simulink library "pil"  (Simulink 3.00)
undefined symbols (not defined in the file or in its folder): j
libraries: smxl x70, SMXL x16
settings Model: LastModifiedBy=campa

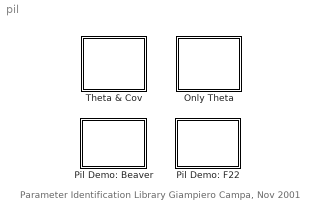
== system pil ==
  note: Parameter Identification Library
      | Giampiero Campa, Nov 2001
  Only Theta : Subsystem
  Pil Demo: Beaver : Subsystem
      settings: OpenFcn=beapilpath=which('pil');path(path,[ beapilpath(1:length(beapilpath)-8) '\examples' ]);clear beapilpath; load beadata; beapil;
      mask Display: disp('Beaver PIL\nDemo')
  Pil Demo: F22 : Subsystem
      settings: OpenFcn=f22pilpath=which('pil');path(path,[ f22pilpath(1:length(f22pilpath)-8) '\examples' ]);clear f22pilpath; load f22data; f22pil;
      mask Display: disp('F22 PIL\nDemo')
  Theta & Cov : Subsystem

== system pil/Only Theta ==
  FTR : Subsystem  mask(Fourier Transform Regression){ths=[4 2], w=2*pi*linspace(0.02,1.8,32)', T=0.025}
      mask prompts: ths "Theta Size"; w "Omega Points"; T "Sample Time"
      mask help:
      | This block performs FTR on the equation :
      |           E*zdot  +  F*z  =  x*TH
      |   The three inputs are respectively x,  E*z, F*z.
      |   The outputs is TH.
      |   The FTR is performed along the points of the omega
      |   vector supplied as the second mask parameter.
      |   The Derivative od E*z is taken by multiplying
      |   its fourier transform by jw.
      mask init:
      | n=length(w);m=ths(1);p=ths(2);
      mask Help:
      | This block performs FTR on the equation :
      |           E*zdot  +  F*z  =  x*TH
      |   The three inputs are respectively x,  E*z, F*z.
      |   The two outputs is TH.
      |   The FTR is performed along the points of the omega
      |   vector supplied as the second mask parameter.
      |   The Derivative od E*z is taken by multiplying
      |   its fourier transform by jw.
      | 
      |   Due to the sampling theorem, for the FT to make
      |   sense the following 2 equations should be valid :
      |   4*pi*wmax*T         <  1 ,
      |   4*pi*Tsim*wmin     >  1 .
      | 
      |   This block needs the Simulink Matrix Library.
  FTR-TD : Subsystem  mask(Fourier Transform Regression (derivative in Time Domain)){ths=[4 2], w=2*pi*linspace(0.02,1.8,32)', T=0.025}
      mask prompts: ths "Theta Size"; w "Omega Points"; T "Sample Time"
      mask help:
      | This block performs FTR on the equation :
      |           E*zdot  +  F*z  =  x*TH
      |   The three inputs are respectively x,  E*z, F*z.
      |   The output is TH.
      |   The FTR is performed along the points of the omega
      |   vector supplied as the second mask parameter.
      |   The Derivative od E*z is taken in the time domain
      |   with the respective simulink block.
      mask init:
      | n=length(w);m=ths(1);p=ths(2);
      mask Help:
      | This block performs FTR on the equation :
      |           E*zdot  +  F*z  =  x*TH
      |   The three inputs are respectively x,  E*z, F*z.
      |   The output is TH.
      |   The FTR is performed along the points of the omega
      |   vector supplied as the second mask parameter.
      |   The Derivative od E*z is taken in the time domain
      |   with the respective simulink block.
      | 
      |   Due to the sampling theorem, for the FT to make
      |   sense the following 2 equations should be valid :
      |   4*pi*wmax*T         <  1 ,
      |   4*pi*Tsim*wmin     >  1 .
      | 
      |   While TH could be of any size, the covariance matrix
      |   is the actual one only if theta is a column vector,
      |   otherwise it's just an approximation of the mean covariance
      |   matrix between the covariance matrices of the different
      |   column vectors that compose TH.
      | 
      |   This block needs the Simulink Matrix Library.
  LLS : Subsystem  mask(Local Least Square){ths=[4 2], n=50, T=0.025}
      mask prompts: ths "Theta Size"; n "Window Size"; T "Sample Time"
      mask help:
      | This block performs LLS on the equation :
      |           E*zdot  +  F*z  =  x*TH
      |   The three inputs are respectively x,  E*z, F*z.
      |   The window size is supplied as a mask parameter.
      mask init:
      | m=ths(1);p=ths(2);
      mask Help:
      | This block performs LLS on the equation :
      |           E*zdot  +  F*z  =  x*TH
      |   The three inputs are respectively x,  E*z, F*z.
      |   The window size is supplied as a mask parameter.
      | 
      |   This block needs the Simulink Matrix Library.
  NRLS : Subsystem  mask(Normalized Recursive Least Squares Regression){ths=[4 2], lam=.9, T=0.025}
      mask prompts: ths "Theta Size"; lam "Forgetting Factor"; T "Sample Time"
      mask help:
      | This block performs NRLS on the equation :
      |           E*zdot  +  F*z  =  x*TH
      |   The three inputs are respectively x,  E*z, F*z.
      |   The outputs is TH.
      |   The forgetting factor is supplied as mask parameter.
      mask init:
      | m=ths(1);p=ths(2);
      mask Help:
      | This block performs RLS on the equation :
      |           E*zdot  +  F*z  =  x*TH
      |   The three inputs are respectively x,  E*z, F*z.
      |   The outputs is TH.
      |   The forgetting factor is supplied as mask parameter.
      | 
      |   This block needs the Simulink Matrix Library.
  RLS : Subsystem  mask(Recursive Least Square Regression){ths=[4 2], lam=.9, T=0.025}
      mask prompts: ths "Theta Size"; lam "Forgetting Factor"; T "Sample Time"
      mask help:
      | This block performs RLS on the equation :
      |           E*zdot  +  F*z  =  x*TH
      |   The three inputs are respectively x,  E*z, F*z.
      |   The outputs is TH.
      |   The forgetting factor is supplied as mask parameter.
      mask init:
      | m=ths(1);p=ths(2);
      mask Help:
      | This block performs RLS on the equation :
      |           E*zdot  +  F*z  =  x*TH
      |   The three inputs are respectively x,  E*z, F*z.
      |   The outputs is TH.
      |   The forgetting factor is supplied as mask parameter.
      | 
      |   This block needs the Simulink Matrix Library.

== system pil/Pil Demo: Beaver ==

== system pil/Pil Demo: F22 ==

== system pil/Theta & Cov ==
  FTR : Subsystem  mask(Fourier Transform Regression){ths=[4 2], w=2*pi*linspace(0.02,1.8,32)', T=0.025}
      mask prompts: ths "Theta Size"; w "Omega Points"; T "Sample Time"
      mask help:
      | This block performs FTR on the equation :
      |           E*zdot  +  F*z  =  x*TH
      |   The three inputs are respectively x,  E*z, F*z.
      |   The two outputs are TH and its covariance matrix.
      |   The FTR is performed along the points of the omega
      |   vector supplied as the second mask parameter.
      |   The Derivative od E*z is taken by multiplying
      |   its fourier transform by jw.
      mask init:
      | n=length(w);m=ths(1);p=ths(2);
      mask Help:
      | This block performs FTR on the equation :
      |           E*zdot  +  F*z  =  x*TH
      |   The three inputs are respectively x,  E*z, F*z.
      |   The two outputs are TH and its covariance matrix.
      |   The FTR is performed along the points of the omega
      |   vector supplied as the second mask parameter.
      |   The Derivative od E*z is taken by multiplying
      |   its fourier transform by jw.
      | 
      |   Due to the sampling theorem, for the FT to make
      |   sense the following 2 equations should be valid :
      |   4*pi*wmax*T         <  1 ,
      |   4*pi*Tsim*wmin     >  1 .
      | 
      |   While TH could be of any size, the covariance matrix
      |   is the actual one only if theta is a column vector,
      |   otherwise it's just an approximation of the mean covariance
      |   matrix between the covariance matrices of the different
      |   column vectors that compose TH.
      | 
      |   This block needs the Simulink Matrix Library.
  FTR-TD : Subsystem  mask(Fourier Transform Regression (derivative in Time Domain)){ths=[4 2], w=2*pi*linspace(0.02,1.8,32)', T=0.025}
      mask prompts: ths "Theta Size"; w "Omega Points"; T "Sample Time"
      mask help:
      | This block performs FTR on the equation :
      |           E*zdot  +  F*z  =  x*TH
      |   The three inputs are respectively x,  E*z, F*z.
      |   The two outputs are TH and its covariance matrix.
      |   The FTR is performed along the points of the omega
      |   vector supplied as the second mask parameter.
      |   The Derivative od E*z is taken in the time domain
      |   with the respective simulink block.
      mask init:
      | n=length(w);m=ths(1);p=ths(2);
      mask Help:
      | This block performs FTR on the equation :
      |           E*zdot  +  F*z  =  x*TH
      |   The three inputs are respectively x,  E*z, F*z.
      |   The two outputs are TH and its covariance matrix.
      |   The FTR is performed along the points of the omega
      |   vector supplied as the second mask parameter.
      |   The Derivative od E*z is taken in the time domain
      |   with the respective simulink block.
      | 
      |   Due to the sampling theorem, for the FT to make
      |   sense the following 2 equations should be valid :
      |   4*pi*wmax*T         <  1 ,
      |   4*pi*Tsim*wmin     >  1 .
      | 
      |   While TH could be of any size, the covariance matrix
      |   is the actual one only if theta is a column vector,
      |   otherwise it's just an approximation of the mean covariance
      |   matrix between the covariance matrices of the different
      |   column vectors that compose TH.
      | 
      |   This block needs the Simulink Matrix Library.
  LWR : Subsystem  mask(Local Weighted Regression){ths=[4 2], n=50, sig=1, T=0.025}
      mask prompts: ths "Theta Size"; n "Window Size"; sig "Gaussian Width"; T "Sample Time"
      mask help:
      | This block performs LWR on the equation :
      |           E*zdot  +  F*z  =  x*TH
      |   The three inputs are respectively x,  E*z, F*z.
      |   The two outputs are TH and its covariance matrix.
      |   The window size and the gaussian width are supplied
      |   as mask parameters. The weighting matrix is diagonal
      |   with W(i,i) = exp(-(x(t)-row(x(t),i))*/(2*sig^2)).
      mask init:
      | m=ths(1);p=ths(2);
      mask Help:
      | This block performs LWR on the equation :
      |           E*zdot  +  F*z  =  x*TH
      |   The three inputs are respectively x,  E*z, F*z.
      |   The two outputs are TH and its covariance matrix.
      |   The window size and the gaussian width are supplied
      |   as mask parameters. The weighting matrix is diagonal
      |   with W(i,i) = exp(-(x(t)-row(x(t),i))*/(2*sig^2)).
      | 
      |   While TH could be of any size, the covariance matrix
      |   is the actual one only if theta is a column vector,
      |   otherwise it's just an approximation of the mean covariance
      |   matrix between the covariance matrices of the different
      |   column vectors that compose TH.
      | 
      |   This block needs the Simulink Matrix Library.
  LWR-RD : Subsystem  mask(Local Weighted Regression with Retention and Deletion){ths=[4 2], n=50, sig=1, Tol=1e-6, x0=1, T=0.025}
      mask prompts: ths "Theta Size"; n "Window Size"; sig "Gaussian Width (sigma)"; Tol "Tolerance (x<tol means x=0)"; x0 "x0 (X0=x0*rand(n,m+2*p))"; T "Sample Time"
      mask help:
      | This block performs LWR on the equation :
      |           E*zdot  +  F*z  =  x*TH
      |   The three inputs are respectively x,  E*z, F*z.
      |   The two outputs are TH and its covariance matrix.
      |   The window size and the gaussian width are supplied
      |   as mask parameters. The weighting matrix is diagonal
      |   with W(i,i) = exp(-(x(t)-row(x(t),i))*/(2*sigma^2)).
      mask init:
      | m=ths(1);p=ths(2);
      mask Help:
      | This block performs LWR on the equation :
      |           E*zdot  +  F*z  =  x*TH
      |   The three inputs are respectively x,  E*z, F*z.
      |   The two outputs are TH and its covariance matrix.
      |   The window size and the gaussian width are supplied
      |   as mask parameters. The weighting matrix is diagonal
      |   with W(i,i) = exp(-(x(t)-row(x(t),i))*/(2*sigma^2)).
      | 
      |   While TH could be of any size, the covariance matrix
      |   is the actual one only if theta is a column vector,
      |   otherwise it's just an approximation of the mean covariance
      |   matrix between the covariance matrices of the different
      |   column vectors that compose TH.
      | 
      |   This block needs the Simulink Matrix Library.
  LWR-RD (Matlab) : Subsystem  mask(Local Weighted Regression with Retention and Deletion){ths=[4 2], n=50, sig=1, Tol=1e-6, T=0.025}
      mask prompts: ths "Theta Size"; n "Window Size"; sig "Gaussian Width (sigma)"; Tol "Tolerance (x<tol means x=0)"; T "Sample Time"
      mask help:
      | This block performs LWR on the equation :
      |           E*zdot  +  F*z  =  x*TH
      |   The three inputs are respectively x,  E*z, F*z.
      |   The two outputs are TH and its covariance matrix.
      |   The window size and the gaussian width are supplied
      |   as mask parameters. The weighting matrix is diagonal
      |   with W(i,i) = exp(-(x(t)-row(x(t),i))*/(2*sigma^2)).
      |   This version is based on the m-file s-function lwrb2.m,
      |   and it is therefore slightly slower than the normal version.
      mask init:
      | m=ths(1);p=ths(2);
      mask Help:
      | This block performs LWR on the equation :
      |           E*zdot  +  F*z  =  x*TH
      |   The three inputs are respectively x,  E*z, F*z.
      |   The two outputs are TH and its covariance matrix.
      |   The window size and the gaussian width are supplied
      |   as mask parameters. The weighting matrix is diagonal
      |   with W(i,i) = exp(-(x(t)-row(x(t),i))*/(2*sigma^2)).
      | 
      |   While TH could be of any size, the covariance matrix
      |   is the actual one only if theta is a column vector,
      |   otherwise it's just an approximation of the mean covariance
      |   matrix between the covariance matrices of the different
      |   column vectors that compose TH.
      | 
      |   This version is based on the m-file s-function lwrb2.m,
      |   and it is therefore slightly slower than the normal version.

== system pil/Only Theta/FTR ==
  x : Inport  Port=1  PortWidth=-1  SampleTime=-1  DataType=auto
      settings: SignalType=auto
  Ez : Inport  Port=2  PortWidth=-1  SampleTime=-1  DataType=auto
      settings: SignalType=auto
  Fz : Inport  Port=3  PortWidth=-1  SampleTime=-1  DataType=auto
      settings: SignalType=auto
  DTFT : Subsystem
  Demux2 : Demux  Outputs=[n*m n*p n*p]
  Mux : Mux  Inputs=[m p p]
  Regression : Subsystem
  Sum4 : Sum  Inputs=|++  SaturateOnIntegerOverflow=on
  jw : Gain  Gain=reshape(j*w*ones(1,p),n*p,1)  SaturateOnIntegerOverflow=on
  Theta : Outport  Port=1
  wires:
  DTFT/1(x(jw)) -> Demux2/1
  Demux2/2 -> jw/1
  Mux/1 -> DTFT/1(x(t))
  x/1 -> Mux/1
  Ez/1 -> Mux/2
  Fz/1 -> Mux/3
  Demux2/1 -> Regression/1(X)
  Demux2/3 -> Sum4/2
  jw/1 -> Sum4/1
  Sum4/1 -> Regression/2(Y)
  Regression/1(Theta) -> Theta/1

== system pil/Only Theta/FTR-TD ==
  x : Inport  Port=1  PortWidth=-1  SampleTime=-1  DataType=auto
      settings: SignalType=auto
  Ez : Inport  Port=2  PortWidth=-1  SampleTime=-1  DataType=auto
      settings: SignalType=auto
  Fz : Inport  Port=3  PortWidth=-1  SampleTime=-1  DataType=auto
      settings: SignalType=auto
  DTFT : Subsystem
  Demux2 : Demux  Outputs=[n*m n*p]
  Gain : Gain  Gain=1/T  SaturateOnIntegerOverflow=on
  Mux : Mux  Inputs=[m p]
  Regression : Subsystem
  Sum5 : Sum  Inputs=+-+  SaturateOnIntegerOverflow=on
  Unit Delay : UnitDelay  X0=zeros(p,1)  SampleTime=T
  Theta : Outport  Port=1
  wires:
  Sum5/1 -> Mux/2
  x/1 -> Mux/1
  Fz/1 -> Sum5/3
  Ez/1 -> Gain/1
  Gain/1 -> Sum5/1, Unit Delay/1
  Unit Delay/1 -> Sum5/2
  Demux2/2 -> Regression/2(Y)
  Demux2/1 -> Regression/1(X)
  Regression/1(Theta) -> Theta/1
  DTFT/1(x(jw)) -> Demux2/1
  Mux/1 -> DTFT/1(x(t))

== system pil/Only Theta/LLS ==
  x : Inport  Port=1  PortWidth=-1  SampleTime=-1  DataType=auto
      settings: SignalType=auto
  Ez : Inport  Port=2  PortWidth=-1  SampleTime=-1  DataType=auto
      settings: SignalType=auto
  Fz : Inport  Port=3  PortWidth=-1  SampleTime=-1  DataType=auto
      settings: SignalType=auto
  1/z Chain : Subsystem  mask(Discrete Time Brunowsky Form){ni=m+p, rd=n-1, x0=0, T=T}
      mask prompts: ni "Number of Inputs"; rd "Number of Delays for each Input"; x0 "Initial Condition"; T "Sample Time"
      mask help: Brunowsky Form System
      mask init:
      | a=[];b=[];c=[];d=[];
      | for i=1:ni,
      | a=[a,zeros(size(a,1),rd);zeros(rd,size(a,2)),diag(ones(rd-1,1),1)];
      | b=[b,zeros(size(b,1),1);zeros(rd,size(b,2)),[zeros(rd-1,1);1]];
      | c=[c,zeros(size(c,1),rd);zeros(rd+1,size(c,2)),[eye(rd);zeros(1,rd)]];
      | d=[d,zeros(size(d,1),1);zeros(rd+1,size(d,2)),[zeros(rd,1);1]];
      | end
      mask Help:
      | <p>
      | This block implements a Brunowsky Form System: every inputs passes through n delays.
      | </p>
      | Outputs are simply all the states of the system.
      mask Display: disp('1/z^n')
  Demux2 : Demux  Outputs=[n*m n*p]
  Gain : Gain  Gain=1/T  SaturateOnIntegerOverflow=on
  Mux : Mux  Inputs=[m p]
  Sum5 : Sum  Inputs=+-+  SaturateOnIntegerOverflow=on
  Unit Delay : UnitDelay  X0=zeros(p,1)  SampleTime=T
  vrmult2 : SMXL/Real Matrices/vrmult  dims=[m n p]
  vrpinv : SMXL/Real Matrices/vrpinv  dims=[n m]  tol=1
  Theta : Outport  Port=1
  wires:
  vrpinv/1 -> vrmult2/1
  vrmult2/1 -> Theta/1
  Mux/1 -> 1/z Chain/1(In)
  Demux2/1 -> vrpinv/1
  Demux2/2 -> vrmult2/2
  1/z Chain/1(Out) -> Demux2/1
  Sum5/1 -> Mux/2
  x/1 -> Mux/1
  Fz/1 -> Sum5/3
  Ez/1 -> Gain/1
  Gain/1 -> Sum5/1, Unit Delay/1
  Unit Delay/1 -> Sum5/2

== system pil/Only Theta/NRLS ==
  x : Inport  Port=1  PortWidth=-1  SampleTime=-1  DataType=auto
      settings: SignalType=auto
  Ez : Inport  Port=2  PortWidth=-1  SampleTime=-1  DataType=auto
      settings: SignalType=auto
  Fz : Inport  Port=3  PortWidth=-1  SampleTime=-1  DataType=auto
      settings: SignalType=auto
  Gain : Gain  Gain=1/T  SaturateOnIntegerOverflow=on
  Regression : Subsystem
  Sum5 : Sum  Inputs=+-+  SaturateOnIntegerOverflow=on
  Unit Delay : UnitDelay  X0=zeros(p,1)  SampleTime=T
  Theta : Outport  Port=1
  wires:
  Regression/1(Theta) -> Theta/1
  Sum5/1 -> Regression/2(Y)
  x/1 -> Regression/1(X)
  Fz/1 -> Sum5/3
  Ez/1 -> Gain/1
  Gain/1 -> Unit Delay/1, Sum5/1
  Unit Delay/1 -> Sum5/2

== system pil/Only Theta/RLS ==
  x : Inport  Port=1  PortWidth=-1  SampleTime=-1  DataType=auto
      settings: SignalType=auto
  Ez : Inport  Port=2  PortWidth=-1  SampleTime=-1  DataType=auto
      settings: SignalType=auto
  Fz : Inport  Port=3  PortWidth=-1  SampleTime=-1  DataType=auto
      settings: SignalType=auto
  Gain : Gain  Gain=1/T  SaturateOnIntegerOverflow=on
  Regression : Subsystem
  Sum5 : Sum  Inputs=+-+  SaturateOnIntegerOverflow=on
  Unit Delay : UnitDelay  X0=zeros(p,1)  SampleTime=T
  Theta : Outport  Port=1
  wires:
  Regression/1(Theta) -> Theta/1
  Sum5/1 -> Regression/2(Y)
  x/1 -> Regression/1(X)
  Fz/1 -> Sum5/3
  Ez/1 -> Gain/1
  Gain/1 -> Sum5/1, Unit Delay/1
  Unit Delay/1 -> Sum5/2

== system pil/Theta & Cov/FTR ==
  x : Inport  Port=1  PortWidth=-1  SampleTime=-1  DataType=auto
      settings: SignalType=auto
  Ez : Inport  Port=2  PortWidth=-1  SampleTime=-1  DataType=auto
      settings: SignalType=auto
  Fz : Inport  Port=3  PortWidth=-1  SampleTime=-1  DataType=auto
      settings: SignalType=auto
  DTFT : Subsystem
  Demux2 : Demux  Outputs=[n*m n*p n*p]
  Mux : Mux  Inputs=[m p p]
  Regression : Subsystem
  Sum4 : Sum  Inputs=|++  SaturateOnIntegerOverflow=on
  jw : Gain  Gain=reshape(j*w*ones(1,p),n*p,1)  SaturateOnIntegerOverflow=on
  Theta : Outport  Port=1
  Cov : Outport  Port=2
  wires:
  DTFT/1(x(jw)) -> Demux2/1
  Demux2/2 -> jw/1
  Mux/1 -> DTFT/1(x(t))
  x/1 -> Mux/1
  Ez/1 -> Mux/2
  Fz/1 -> Mux/3
  Demux2/1 -> Regression/1(X)
  Demux2/3 -> Sum4/2
  jw/1 -> Sum4/1
  Sum4/1 -> Regression/2(Y)
  Regression/1(Theta) -> Theta/1
  Regression/2(Cov) -> Cov/1

== system pil/Theta & Cov/FTR-TD ==
  x : Inport  Port=1  PortWidth=-1  SampleTime=-1  DataType=auto
      settings: SignalType=auto
  Ez : Inport  Port=2  PortWidth=-1  SampleTime=-1  DataType=auto
      settings: SignalType=auto
  Fz : Inport  Port=3  PortWidth=-1  SampleTime=-1  DataType=auto
      settings: SignalType=auto
  DTFT : Subsystem
  Demux2 : Demux  Outputs=[n*m n*p]
  Gain : Gain  Gain=1/T  SaturateOnIntegerOverflow=on
  Mux : Mux  Inputs=[m p]
  Regression : Subsystem
  Sum5 : Sum  Inputs=+-+  SaturateOnIntegerOverflow=on
  Unit Delay : UnitDelay  X0=zeros(p,1)  SampleTime=T
  Theta : Outport  Port=1
  Cov : Outport  Port=2
  wires:
  DTFT/1(x(jw)) -> Demux2/1
  Regression/2(Cov) -> Cov/1
  Regression/1(Theta) -> Theta/1
  Demux2/1 -> Regression/1(X)
  Demux2/2 -> Regression/2(Y)
  Sum5/1 -> Mux/2
  x/1 -> Mux/1
  Fz/1 -> Sum5/3
  Ez/1 -> Gain/1
  Gain/1 -> Unit Delay/1, Sum5/1
  Unit Delay/1 -> Sum5/2
  Mux/1 -> DTFT/1(x(t))

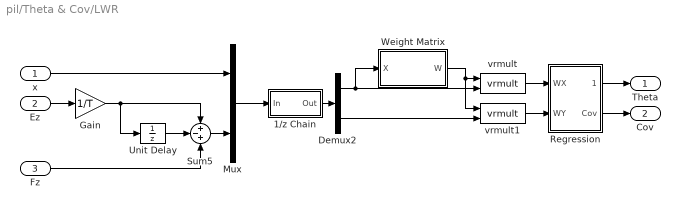
== system pil/Theta & Cov/LWR ==
  x : Inport  Port=1  PortWidth=-1  SampleTime=-1  DataType=auto
      settings: SignalType=auto
  Ez : Inport  Port=2  PortWidth=-1  SampleTime=-1  DataType=auto
      settings: SignalType=auto
  Fz : Inport  Port=3  PortWidth=-1  SampleTime=-1  DataType=auto
      settings: SignalType=auto
  1/z Chain : Subsystem  mask(Discrete Time Brunowsky Form){ni=m+p, rd=n-1, x0=0, T=T}
      mask prompts: ni "Number of Inputs"; rd "Number of Delays for each Input"; x0 "Initial Condition"; T "Sample Time"
      mask help: Brunowsky Form System
      mask init: same as pil/Only Theta/LLS/1/z Chain
      mask Help:
      | <p>
      | This block implements a Brunowsky Form System: every inputs passes through n delays.
      | </p>
      | Outputs are simply all the states of the system.
      mask Display: disp('1/z^n')
  Demux2 : Demux  Outputs=[n*m n*p]
  Gain : Gain  Gain=1/T  SaturateOnIntegerOverflow=on
  Mux : Mux  Inputs=[m p]
  Regression : Subsystem
  Sum5 : Sum  Inputs=+-+  SaturateOnIntegerOverflow=on
  Unit Delay : UnitDelay  X0=zeros(p,1)  SampleTime=T
  Weight Matrix : Subsystem
  vrmult : SMXL/Real Matrices/vrmult  dims=[n n m]
  vrmult1 : SMXL/Real Matrices/vrmult  dims=[n n p]
  Theta : Outport  Port=1
  Cov : Outport  Port=2
  wires:
  Sum5/1 -> Mux/2
  x/1 -> Mux/1
  Fz/1 -> Sum5/3
  Gain/1 -> Unit Delay/1, Sum5/1
  Unit Delay/1 -> Sum5/2
  Ez/1 -> Gain/1
  1/z Chain/1(Out) -> Demux2/1
  Regression/1(Theta) -> Theta/1
  vrmult1/1 -> Regression/2(WY)
  vrmult/1 -> Regression/1(WX)
  Weight Matrix/1(W) -> vrmult1/1, vrmult/1
  Demux2/1 -> vrmult/2, Weight Matrix/1(X)
  Regression/2(Cov) -> Cov/1
  Demux2/2 -> vrmult1/2
  Mux/1 -> 1/z Chain/1(In)

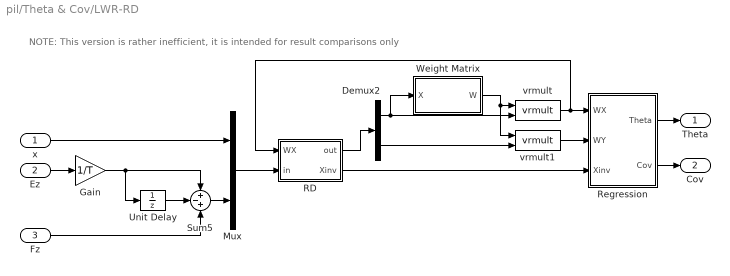
== system pil/Theta & Cov/LWR-RD ==
  note: NOTE: This version is rather inefficient, it is intended for result comparisons only
  x : Inport  Port=1  PortWidth=-1  SampleTime=-1  DataType=auto
      settings: SignalType=auto
  Ez : Inport  Port=2  PortWidth=-1  SampleTime=-1  DataType=auto
      settings: SignalType=auto
  Fz : Inport  Port=3  PortWidth=-1  SampleTime=-1  DataType=auto
      settings: SignalType=auto
  Demux2 : Demux  Outputs=[n*m n*p]
  Gain : Gain  Gain=1/T  SaturateOnIntegerOverflow=on
  Mux : Mux  Inputs=[m p]
  RD : Subsystem
  Regression : Subsystem
  Sum5 : Sum  Inputs=+-+  SaturateOnIntegerOverflow=on
  Unit Delay : UnitDelay  X0=zeros(p,1)  SampleTime=T
  Weight Matrix : Subsystem
  vrmult : smxl/Real Matrices/vrmult  dims=[n n m]
  vrmult1 : smxl/Real Matrices/vrmult  dims=[n n p]
  Theta : Outport  Port=1
  Cov : Outport  Port=2
  wires:
  Regression/2(Cov) -> Cov/1
  vrmult/1 -> RD/1(WX), Regression/1(WX)
  Weight Matrix/1(W) -> vrmult/1, vrmult1/1
  vrmult1/1 -> Regression/2(WY)
  Regression/1(Theta) -> Theta/1
  RD/1(out) -> Demux2/1
  Demux2/1 -> Weight Matrix/1(X), vrmult/2
  Demux2/2 -> vrmult1/2
  RD/2(Xinv) -> Regression/3(Xinv)
  Sum5/1 -> Mux/2
  x/1 -> Mux/1
  Fz/1 -> Sum5/3
  Gain/1 -> Sum5/1, Unit Delay/1
  Unit Delay/1 -> Sum5/2
  Ez/1 -> Gain/1
  Mux/1 -> RD/2(in)

== system pil/Theta & Cov/LWR-RD (Matlab) ==
  note: Matlab Version of the Boeing LWR/RD code
  x : Inport  Port=1  PortWidth=-1  SampleTime=-1  DataType=auto
      settings: SignalType=auto
  Ez : Inport  Port=2  PortWidth=-1  SampleTime=-1  DataType=auto
      settings: SignalType=auto
  Fz : Inport  Port=3  PortWidth=-1  SampleTime=-1  DataType=auto
      settings: SignalType=auto
  Demux : Demux  Outputs=[m*p m*m]
  Gain : Gain  Gain=1/T  SaturateOnIntegerOverflow=on
  Mux : Mux  Inputs=[m p]
  S-Function : S-Function  FunctionName=lwrb2  Parameters=n,m,p,sig,Tol,T  PortCounts=[]  SFunctionModules=''
  Sum5 : Sum  Inputs=+-+  SaturateOnIntegerOverflow=on
  Unit Delay : UnitDelay  X0=zeros(p,1)  SampleTime=T
  Theta : Outport  Port=1
  Cov : Outport  Port=2
  wires:
  Mux/1 -> S-Function/1
  Sum5/1 -> Mux/2
  x/1 -> Mux/1
  Fz/1 -> Sum5/3
  Gain/1 -> Unit Delay/1, Sum5/1
  Unit Delay/1 -> Sum5/2
  Ez/1 -> Gain/1
  S-Function/1 -> Demux/1
  Demux/1 -> Theta/1
  Demux/2 -> Cov/1

== system pil/Only Theta/FTR/DTFT ==
  x(t) : Inport  Port=1  PortWidth=-1  SampleTime=-1  DataType=auto
      settings: SignalType=auto
  -j*w : Constant  Value=-j*w
  Math Function : Math  Operator=exp  OutputSignalType=complex
  Product : Product  Inputs=2  SaturateOnIntegerOverflow=on
  Sum1 : Sum  Inputs=|++  SaturateOnIntegerOverflow=on
  Unit Delay1 : UnitDelay  Orientation=left  X0=zeros(n*(m+2*p),1)  SampleTime=T
  k*dt : DigitalClock  SampleTime=T
  vcmult22 : smxl/Complex Matrices/vcmult  d=[n 1 (m+2*p)]
  x(jw) : Outport  Port=1
  wires:
  vcmult22/1 -> Sum1/1
  Unit Delay1/1 -> Sum1/2
  Math Function/1 -> vcmult22/1
  Product/1 -> Math Function/1
  Sum1/1 -> Unit Delay1/1, x(jw)/1
  x(t)/1 -> vcmult22/2
  -j*w/1 -> Product/2
  k*dt/1 -> Product/1

== system pil/Only Theta/FTR/Regression ==
  note: Th=Xinv*real(X'*Y);
  note: Xinv=inv(real(X'*X));
  X : Inport  Port=1  PortWidth=-1  SampleTime=-1  DataType=auto
      settings: SignalType=auto
  Y : Inport  Port=2  PortWidth=-1  SampleTime=-1  DataType=auto
      settings: SignalType=auto
  Complex to Real-Imag : ComplexToRealImag  Output=RealAndImag
  Complex to Real-Imag2 : ComplexToRealImag  Output=RealAndImag
  Terminator : Terminator
  Terminator3 : Terminator
  vcmult16 : smxl/Complex Matrices/vcmult  d=[m n p]
  vcmult3 : smxl/Complex Matrices/vcmult  d=[m n m]
  vctrsp : smxl/Complex Matrices/vctrsp  d=[n m]  h=on
  vrmult : smxl/Real Matrices/vrmult  dims=[m m p]
  vrpinv : smxl/Real Matrices/vrpinv  dims=[m m]  tol=1
  Theta : Outport  Port=1
  wires:
  vrmult/1 -> Theta/1
  Y/1 -> vcmult16/2
  vrpinv/1 -> vrmult/1
  vctrsp/1 -> vcmult16/1, vcmult3/1
  X/1 -> vcmult3/2, vctrsp/1
  vcmult3/1 -> Complex to Real-Imag/1
  Complex to Real-Imag/2 -> Terminator/1
  Complex to Real-Imag/1 -> vrpinv/1
  Complex to Real-Imag2/2 -> Terminator3/1
  Complex to Real-Imag2/1 -> vrmult/2
  vcmult16/1 -> Complex to Real-Imag2/1

== system pil/Only Theta/FTR-TD/DTFT ==
  x(t) : Inport  Port=1  PortWidth=-1  SampleTime=-1  DataType=auto
      settings: SignalType=auto
  -j*w : Constant  Value=-j*w
  Math Function : Math  Operator=exp  OutputSignalType=complex
  Product : Product  Inputs=2  SaturateOnIntegerOverflow=on
  Sum1 : Sum  Inputs=|++  SaturateOnIntegerOverflow=on
  Unit Delay1 : UnitDelay  Orientation=left  X0=zeros(n*(m+p),1)  SampleTime=T
  k*dt : DigitalClock  SampleTime=T
  vcmult22 : smxl/Complex Matrices/vcmult  d=[n 1 (m+p)]
  x(jw) : Outport  Port=1
  wires:
  vcmult22/1 -> Sum1/1
  Unit Delay1/1 -> Sum1/2
  Math Function/1 -> vcmult22/1
  Product/1 -> Math Function/1
  Sum1/1 -> Unit Delay1/1, x(jw)/1
  x(t)/1 -> vcmult22/2
  -j*w/1 -> Product/2
  k*dt/1 -> Product/1

== system pil/Only Theta/FTR-TD/Regression ==
  note: Xinv=inv(real(X'*X));
  X : Inport  Port=1  PortWidth=-1  SampleTime=-1  DataType=auto
      settings: SignalType=auto
  Y : Inport  Port=2  PortWidth=-1  SampleTime=-1  DataType=auto
      settings: SignalType=auto
  Complex to Real-Imag : ComplexToRealImag  Output=RealAndImag
  Complex to Real-Imag2 : ComplexToRealImag  Output=RealAndImag
  Terminator : Terminator
  Terminator3 : Terminator
  vcmult16 : smxl/Complex Matrices/vcmult  d=[m n p]
  vcmult3 : smxl/Complex Matrices/vcmult  d=[m n m]
  vctrsp : smxl/Complex Matrices/vctrsp  d=[n m]  h=on
  vrmult : smxl/Real Matrices/vrmult  dims=[m m p]
  vrpinv : smxl/Real Matrices/vrpinv  dims=[m m]  tol=1
  Theta : Outport  Port=1
  wires:
  vctrsp/1 -> vcmult16/1, vcmult3/1
  X/1 -> vcmult3/2, vctrsp/1
  vcmult3/1 -> Complex to Real-Imag/1
  Complex to Real-Imag/2 -> Terminator/1
  Complex to Real-Imag/1 -> vrpinv/1
  Complex to Real-Imag2/2 -> Terminator3/1
  Complex to Real-Imag2/1 -> vrmult/2
  vcmult16/1 -> Complex to Real-Imag2/1
  vrmult/1 -> Theta/1
  vrpinv/1 -> vrmult/1
  Y/1 -> vcmult16/2

== system pil/Only Theta/LLS/1/z Chain ==
  In : Inport  Port=1  PortWidth=-1  SampleTime=-1  DataType=auto
      settings: SignalType=auto
  Discrete State-Space : DiscreteStateSpace  A=a  B=b  C=c  D=d  X0=x0  SampleTime=T
  Out : Outport  Port=1
  wires:
  In/1 -> Discrete State-Space/1
  Discrete State-Space/1 -> Out/1

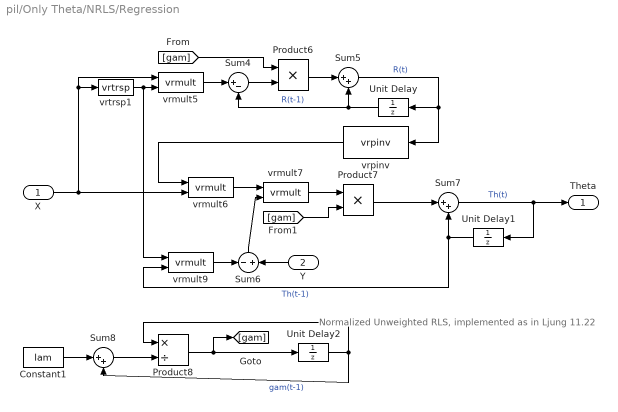
== system pil/Only Theta/NRLS/Regression ==
  note: Normalized Unweighted RLS,
      |  implemented as in Ljung 11.22
  X : Inport  Port=1  PortWidth=-1  SampleTime=-1  DataType=auto
      settings: SignalType=auto
  Y : Inport  Orientation=left  Port=2  PortWidth=-1  SampleTime=-1  DataType=auto
      settings: SignalType=auto
  Constant1 : Constant  Value=lam
  Product6 : Product  Inputs=2  SaturateOnIntegerOverflow=on
  Product7 : Product  Inputs=2  SaturateOnIntegerOverflow=on
  Product8 : Product  Inputs=*/  SaturateOnIntegerOverflow=on
  Sum4 : Sum  Inputs=|+-  SaturateOnIntegerOverflow=on
  Sum5 : Sum  Inputs=|++  SaturateOnIntegerOverflow=on
  Sum6 : Sum  Orientation=up  Inputs=-|+  SaturateOnIntegerOverflow=on
  Sum7 : Sum  Inputs=|++  SaturateOnIntegerOverflow=on
  Sum8 : Sum  Inputs=|++  SaturateOnIntegerOverflow=on
  Unit Delay : UnitDelay  Orientation=left  X0=eps*reshape(eye(m),m^2,1)  SampleTime=T
  Unit Delay1 : UnitDelay  Orientation=left  X0=0  SampleTime=T
  Unit Delay2 : UnitDelay  X0=1  SampleTime=T
  vrmult5 : SMXL/Real Matrices/vrmult  dims=[m 1 m]
  vrmult6 : SMXL/Real Matrices/vrmult  dims=[m m 1]
  vrmult7 : SMXL/Real Matrices/vrmult  dims=[m 1 p]
  vrmult9 : SMXL/Real Matrices/vrmult  dims=[1 m p]
  vrpinv : SMXL/Real Matrices/vrpinv  Orientation=left  dims=[m m]  tol=1
  vrtrsp1 : SMXL/Real Matrices/vrtrsp  dims=[m 1]
  Theta : Outport  Port=1
  wires:
  Product8/1 -> [gam], Unit Delay2/1
  Unit Delay2/1 -> Product8/1, Sum8/2  "gam(t-1)"
  Sum8/1 -> Product8/2
  Constant1/1 -> Sum8/1
  [gam] -> Product7/2
  [gam] -> Product6/1
  Unit Delay1/1 -> vrmult9/2, Sum7/2  "Th(t-1)"
  Sum7/1 -> Theta/1, Unit Delay1/1  "Th(t)"
  Product7/1 -> Sum7/1
  vrmult7/1 -> Product7/1
  vrmult9/1 -> Sum6/1
  vrtrsp1/1 -> vrmult9/1, vrmult5/2
  Y/1 -> Sum6/2
  Sum6/1 -> vrmult7/2
  vrmult6/1 -> vrmult7/1
  X/1 -> vrmult6/2, vrmult5/1, vrtrsp1/1
  vrpinv/1 -> vrmult6/1
  Sum5/1 -> vrpinv/1, Unit Delay/1  "R(t)"
  Unit Delay/1 -> Sum5/2, Sum4/2  "R(t-1)"
  Product6/1 -> Sum5/1
  Sum4/1 -> Product6/2
  vrmult5/1 -> Sum4/1

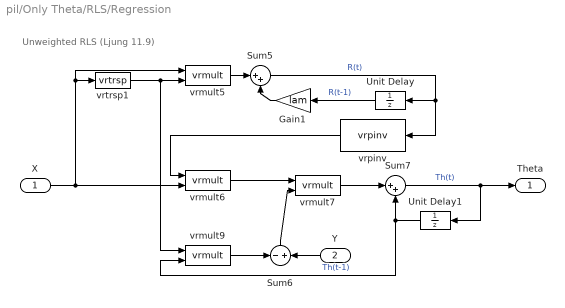
== system pil/Only Theta/RLS/Regression ==
  note: Unweighted RLS (Ljung 11.9)
  X : Inport  Port=1  PortWidth=-1  SampleTime=-1  DataType=auto
      settings: SignalType=auto
  Y : Inport  Orientation=left  Port=2  PortWidth=-1  SampleTime=-1  DataType=auto
      settings: SignalType=auto
  Gain1 : Gain  Orientation=left  Gain=lam  SaturateOnIntegerOverflow=on
  Sum5 : Sum  Inputs=|++  SaturateOnIntegerOverflow=on
  Sum6 : Sum  Orientation=up  Inputs=-|+  SaturateOnIntegerOverflow=on
  Sum7 : Sum  Inputs=|++  SaturateOnIntegerOverflow=on
  Unit Delay : UnitDelay  Orientation=left  X0=eps*reshape(eye(m),m^2,1)  SampleTime=T
  Unit Delay1 : UnitDelay  Orientation=left  X0=0  SampleTime=T
  vrmult5 : SMXL/Real Matrices/vrmult  dims=[m 1 m]
  vrmult6 : SMXL/Real Matrices/vrmult  dims=[m m 1]
  vrmult7 : SMXL/Real Matrices/vrmult  dims=[m 1 p]
  vrmult9 : SMXL/Real Matrices/vrmult  dims=[1 m p]
  vrpinv : SMXL/Real Matrices/vrpinv  Orientation=left  dims=[m m]  tol=1
  vrtrsp1 : SMXL/Real Matrices/vrtrsp  dims=[m 1]
  Theta : Outport  Port=1
  wires:
  Sum5/1 -> vrpinv/1, Unit Delay/1  "R(t)"
  Sum6/1 -> vrmult7/2
  Y/1 -> Sum6/2
  Gain1/1 -> Sum5/2
  Unit Delay/1 -> Gain1/1  "R(t-1)"
  Unit Delay1/1 -> vrmult9/2, Sum7/2  "Th(t-1)"
  Sum7/1 -> Theta/1, Unit Delay1/1  "Th(t)"
  vrmult7/1 -> Sum7/1
  vrmult6/1 -> vrmult7/1
  vrmult9/1 -> Sum6/1
  vrtrsp1/1 -> vrmult9/1, vrmult5/2
  X/1 -> vrmult6/2, vrmult5/1, vrtrsp1/1
  vrpinv/1 -> vrmult6/1
  vrmult5/1 -> Sum5/1

== system pil/Theta & Cov/FTR/DTFT ==
  x(t) : Inport  Port=1  PortWidth=-1  SampleTime=-1  DataType=auto
      settings: SignalType=auto
  -j*w : Constant  Value=-j*w
  Math Function : Math  Operator=exp  OutputSignalType=complex
  Product : Product  Inputs=2  SaturateOnIntegerOverflow=on
  Sum1 : Sum  Inputs=|++  SaturateOnIntegerOverflow=on
  Unit Delay1 : UnitDelay  Orientation=left  X0=zeros(n*(m+2*p),1)  SampleTime=T
  k*dt : DigitalClock  SampleTime=T
  vcmult22 : smxl/Complex Matrices/vcmult  d=[n 1 (m+2*p)]
  x(jw) : Outport  Port=1
  wires:
  vcmult22/1 -> Sum1/1
  Unit Delay1/1 -> Sum1/2
  Math Function/1 -> vcmult22/1
  Product/1 -> Math Function/1
  Sum1/1 -> Unit Delay1/1, x(jw)/1
  x(t)/1 -> vcmult22/2
  -j*w/1 -> Product/2
  k*dt/1 -> Product/1

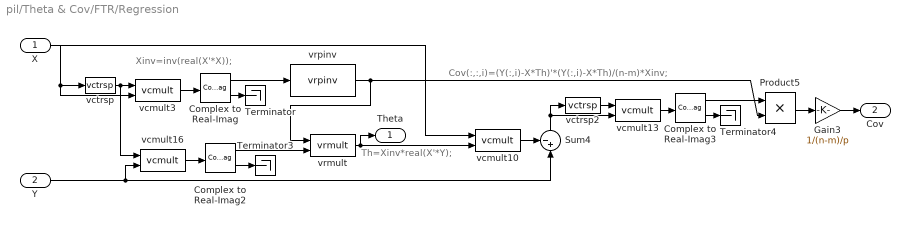
== system pil/Theta & Cov/FTR/Regression ==
  note: Th=Xinv*real(X'*Y);
  note: Cov(:,:,i)=(Y(:,i)-X*Th)'*(Y(:,i)-X*Th)/(n-m)*Xinv;
  note: Xinv=inv(real(X'*X));
  X : Inport  Port=1  PortWidth=-1  SampleTime=-1  DataType=auto
      settings: SignalType=auto
  Y : Inport  Port=2  PortWidth=-1  SampleTime=-1  DataType=auto
      settings: SignalType=auto
  Complex to Real-Imag : ComplexToRealImag  Output=RealAndImag
  Complex to Real-Imag2 : ComplexToRealImag  Output=RealAndImag
  Complex to Real-Imag3 : ComplexToRealImag  Output=RealAndImag
  Gain3 : Gain  Gain=1/(n-m)/p  SaturateOnIntegerOverflow=on
  Product5 : Product  Inputs=2  SaturateOnIntegerOverflow=on
  Sum4 : Sum  Orientation=up  Inputs=-+|  SaturateOnIntegerOverflow=on
  Terminator : Terminator
  Terminator3 : Terminator
  Terminator4 : Terminator
  vcmult10 : smxl/Complex Matrices/vcmult  d=[n m p]
  vcmult13 : smxl/Complex Matrices/vcmult  d=[1 n*p 1]
  vcmult16 : smxl/Complex Matrices/vcmult  d=[m n p]
  vcmult3 : smxl/Complex Matrices/vcmult  d=[m n m]
  vctrsp : smxl/Complex Matrices/vctrsp  d=[n m]  h=on
  vctrsp2 : smxl/Complex Matrices/vctrsp  d=[n*p 1]  h=on
  vrmult : smxl/Real Matrices/vrmult  dims=[m m p]
  vrpinv : smxl/Real Matrices/vrpinv  dims=[m m]  tol=1
  Theta : Outport  Port=1
  Cov : Outport  Port=2
  wires:
  vctrsp/1 -> vcmult16/1, vcmult3/1
  X/1 -> vcmult3/2, vctrsp/1, vcmult10/1
  vcmult3/1 -> Complex to Real-Imag/1
  Complex to Real-Imag/2 -> Terminator/1
  Complex to Real-Imag/1 -> vrpinv/1
  vrpinv/1 -> Product5/2, vrmult/1
  Complex to Real-Imag2/2 -> Terminator3/1
  Complex to Real-Imag2/1 -> vrmult/2
  vcmult16/1 -> Complex to Real-Imag2/1
  Y/1 -> vcmult16/2, Sum4/2
  vcmult10/1 -> Sum4/1
  vrmult/1 -> vcmult10/2, Theta/1
  vctrsp2/1 -> vcmult13/1
  Sum4/1 -> vctrsp2/1, vcmult13/2
  vcmult13/1 -> Complex to Real-Imag3/1
  Complex to Real-Imag3/2 -> Terminator4/1
  Product5/1 -> Gain3/1
  Gain3/1 -> Cov/1
  Complex to Real-Imag3/1 -> Product5/1

== system pil/Theta & Cov/FTR-TD/DTFT ==
  x(t) : Inport  Port=1  PortWidth=-1  SampleTime=-1  DataType=auto
      settings: SignalType=auto
  -j*w : Constant  Value=-j*w
  Math Function : Math  Operator=exp  OutputSignalType=complex
  Product : Product  Inputs=2  SaturateOnIntegerOverflow=on
  Sum1 : Sum  Inputs=|++  SaturateOnIntegerOverflow=on
  Unit Delay1 : UnitDelay  Orientation=left  X0=zeros(n*(m+p),1)  SampleTime=T
  k*dt : DigitalClock  SampleTime=T
  vcmult22 : smxl/Complex Matrices/vcmult  d=[n 1 (m+p)]
  x(jw) : Outport  Port=1
  wires:
  k*dt/1 -> Product/1
  -j*w/1 -> Product/2
  x(t)/1 -> vcmult22/2
  Sum1/1 -> x(jw)/1, Unit Delay1/1
  Product/1 -> Math Function/1
  Math Function/1 -> vcmult22/1
  Unit Delay1/1 -> Sum1/2
  vcmult22/1 -> Sum1/1

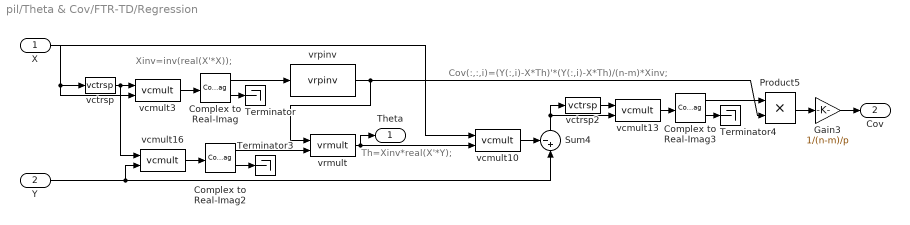
== system pil/Theta & Cov/FTR-TD/Regression ==
  note: Xinv=inv(real(X'*X));
  note: Cov(:,:,i)=(Y(:,i)-X*Th)'*(Y(:,i)-X*Th)/(n-m)*Xinv;
  note: Th=Xinv*real(X'*Y);
  X : Inport  Port=1  PortWidth=-1  SampleTime=-1  DataType=auto
      settings: SignalType=auto
  Y : Inport  Port=2  PortWidth=-1  SampleTime=-1  DataType=auto
      settings: SignalType=auto
  Complex to Real-Imag : ComplexToRealImag  Output=RealAndImag
  Complex to Real-Imag2 : ComplexToRealImag  Output=RealAndImag
  Complex to Real-Imag3 : ComplexToRealImag  Output=RealAndImag
  Gain3 : Gain  Gain=1/(n-m)/p  SaturateOnIntegerOverflow=on
  Product5 : Product  Inputs=2  SaturateOnIntegerOverflow=on
  Sum4 : Sum  Orientation=up  Inputs=-+|  SaturateOnIntegerOverflow=on
  Terminator : Terminator
  Terminator3 : Terminator
  Terminator4 : Terminator
  vcmult10 : smxl/Complex Matrices/vcmult  d=[n m p]
  vcmult13 : smxl/Complex Matrices/vcmult  d=[1 n*p 1]
  vcmult16 : smxl/Complex Matrices/vcmult  d=[m n p]
  vcmult3 : smxl/Complex Matrices/vcmult  d=[m n m]
  vctrsp : smxl/Complex Matrices/vctrsp  d=[n m]  h=on
  vctrsp2 : smxl/Complex Matrices/vctrsp  d=[n*p 1]  h=on
  vrmult : smxl/Real Matrices/vrmult  dims=[m m p]
  vrpinv : smxl/Real Matrices/vrpinv  dims=[m m]  tol=1
  Theta : Outport  Port=1
  Cov : Outport  Port=2
  wires:
  Complex to Real-Imag3/1 -> Product5/1
  Gain3/1 -> Cov/1
  Product5/1 -> Gain3/1
  Complex to Real-Imag3/2 -> Terminator4/1
  vcmult13/1 -> Complex to Real-Imag3/1
  Sum4/1 -> vcmult13/2, vctrsp2/1
  vctrsp2/1 -> vcmult13/1
  vrmult/1 -> Theta/1, vcmult10/2
  vcmult10/1 -> Sum4/1
  Y/1 -> Sum4/2, vcmult16/2
  vcmult16/1 -> Complex to Real-Imag2/1
  Complex to Real-Imag2/1 -> vrmult/2
  Complex to Real-Imag2/2 -> Terminator3/1
  vrpinv/1 -> vrmult/1, Product5/2
  Complex to Real-Imag/1 -> vrpinv/1
  Complex to Real-Imag/2 -> Terminator/1
  vcmult3/1 -> Complex to Real-Imag/1
  X/1 -> vcmult10/1, vctrsp/1, vcmult3/2
  vctrsp/1 -> vcmult3/1, vcmult16/1

== system pil/Theta & Cov/LWR/1/z Chain ==
  In : Inport  Port=1  PortWidth=-1  SampleTime=-1  DataType=auto
      settings: SignalType=auto
  Discrete State-Space : DiscreteStateSpace  A=a  B=b  C=c  D=d  X0=x0  SampleTime=T
  Out : Outport  Port=1
  wires:
  Discrete State-Space/1 -> Out/1
  In/1 -> Discrete State-Space/1

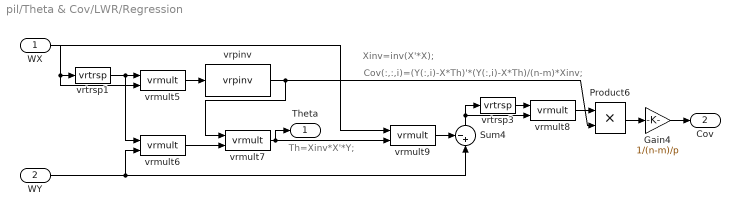
== system pil/Theta & Cov/LWR/Regression ==
  note: Xinv=inv(X'*X);
  note: Th=Xinv*X'*Y;
  note: Cov(:,:,i)=(Y(:,i)-X*Th)'*(Y(:,i)-X*Th)/(n-m)*Xinv;
  WX : Inport  Port=1  PortWidth=-1  SampleTime=-1  DataType=auto
      settings: SignalType=auto
  WY : Inport  Port=2  PortWidth=-1  SampleTime=-1  DataType=auto
      settings: SignalType=auto
  Gain4 : Gain  Gain=1/(n-m)/p  SaturateOnIntegerOverflow=on
  Product6 : Product  Inputs=2  SaturateOnIntegerOverflow=on
  Sum4 : Sum  Orientation=up  Inputs=-+|  SaturateOnIntegerOverflow=on
  vrmult5 : smxl/Real Matrices/vrmult  dims=[m n m]
  vrmult6 : smxl/Real Matrices/vrmult  dims=[m n p]
  vrmult7 : smxl/Real Matrices/vrmult  dims=[m m p]
  vrmult8 : smxl/Real Matrices/vrmult  dims=[1 n*p 1]
  vrmult9 : smxl/Real Matrices/vrmult  dims=[n m p]
  vrpinv : smxl/Real Matrices/vrpinv  dims=[m m]  tol=1
  vrtrsp1 : smxl/Real Matrices/vrtrsp  dims=[n m]
  vrtrsp3 : smxl/Real Matrices/vrtrsp  dims=[n*p 1]
  Theta : Outport  Port=1
  Cov : Outport  Port=2
  wires:
  vrtrsp1/1 -> vrmult6/1, vrmult5/1
  vrmult6/1 -> vrmult7/2
  vrmult9/1 -> Sum4/1
  vrmult7/1 -> Theta/1, vrmult9/2
  Sum4/1 -> vrmult8/2, vrtrsp3/1
  vrmult8/1 -> Product6/1
  Product6/1 -> Gain4/1
  Gain4/1 -> Cov/1
  vrpinv/1 -> vrmult7/1, Product6/2
  vrtrsp3/1 -> vrmult8/1
  WY/1 -> Sum4/2, vrmult6/2
  vrmult5/1 -> vrpinv/1
  WX/1 -> vrmult5/2, vrmult9/1, vrtrsp1/1

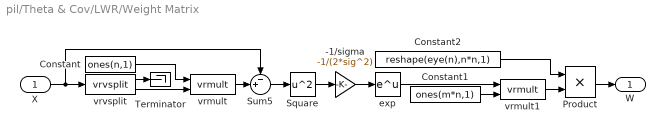
== system pil/Theta & Cov/LWR/Weight Matrix ==
  X : Inport  Port=1  PortWidth=-1  SampleTime=-1  DataType=auto
      settings: SignalType=auto
  -1/sigma : Gain  Gain=-1/(2*sig^2)  SaturateOnIntegerOverflow=on
  Constant : Constant  Value=ones(n,1)
  Constant1 : Constant  Value=ones(m*n,1)
  Constant2 : Constant  Value=reshape(eye(n),n*n,1)
  Product : Product  Inputs=2  SaturateOnIntegerOverflow=on
  Square : Math  Operator=square  OutputSignalType=auto
  Sum5 : Sum  Inputs=-+|  SaturateOnIntegerOverflow=on
  Terminator : Terminator
  exp : Math  Operator=exp  OutputSignalType=auto
  vrmult : smxl/Real Matrices/vrmult  dims=[n 1 m]
  vrmult1 : smxl/Real Matrices/vrmult  dims=[n m n]
  vrvsplit : smxl/Real Matrices/vrvsplit  dims=[n-1 1 m]
  W : Outport  Port=1
  wires:
  exp/1 -> vrmult1/1
  Constant1/1 -> vrmult1/2
  vrmult1/1 -> Product/2
  Constant2/1 -> Product/1
  Product/1 -> W/1
  -1/sigma/1 -> exp/1
  Square/1 -> -1/sigma/1
  vrmult/1 -> Sum5/2
  Constant/1 -> vrmult/1
  Sum5/1 -> Square/1
  vrvsplit/2 -> vrmult/2
  vrvsplit/1 -> Terminator/1
  X/1 -> Sum5/1, vrvsplit/1

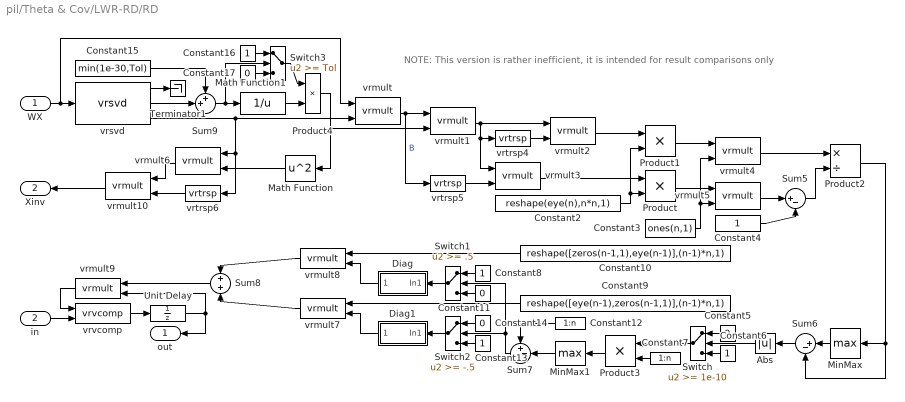
== system pil/Theta & Cov/LWR-RD/RD ==
  note: NOTE: This version is rather inefficient, it is intended for result comparisons only
  WX : Inport  Port=1  PortWidth=-1  SampleTime=-1  DataType=auto
      settings: SignalType=auto
  in : Inport  Port=2  PortWidth=-1  SampleTime=-1  DataType=auto
      settings: SignalType=auto
  Abs : Abs  Orientation=left
  Constant10 : Constant  Orientation=left  Value=reshape([zeros(n-1,1),eye(n-1)],(n-1)*n,1)
  Constant11 : Constant  Orientation=left  Value=0
  Constant12 : Constant  Orientation=left  Value=1:n
  Constant13 : Constant  Orientation=left  Value=1
  Constant14 : Constant  Orientation=left  Value=0
  Constant15 : Constant  Value=min(1e-30,Tol)
  Constant16 : Constant  Value=1
  Constant17 : Constant  Value=0
  Constant2 : Constant  Value=reshape(eye(n),n*n,1)
  Constant3 : Constant  Value=ones(n,1)
  Constant4 : Constant  Value=1
  Constant5 : Constant  Orientation=left  Value=0
  Constant6 : Constant  Orientation=left  Value=1
  Constant7 : Constant  Orientation=left  Value=1:n
  Constant8 : Constant  Orientation=left  Value=1
  Constant9 : Constant  Orientation=left  Value=reshape([eye(n-1),zeros(n-1,1)],(n-1)*n,1)
  Diag : Subsystem  Orientation=left
  Diag1 : Subsystem  Orientation=left
  Math Function : Math  Orientation=left  Operator=square  OutputSignalType=auto
  Math Function1 : Math  Operator=reciprocal  OutputSignalType=auto
  MinMax : MinMax  Orientation=left  Function=max  Inputs=1
  MinMax1 : MinMax  Orientation=left  Function=max  Inputs=1
  Product : Product  Inputs=2  SaturateOnIntegerOverflow=on
  Product1 : Product  Inputs=2  SaturateOnIntegerOverflow=on
  Product2 : Product  Inputs=*/  SaturateOnIntegerOverflow=on
  Product3 : Product  Orientation=left  Inputs=2  SaturateOnIntegerOverflow=on
  Product4 : Product  Inputs=2  SaturateOnIntegerOverflow=on
  Sum5 : Sum  Inputs=|+-  SaturateOnIntegerOverflow=on
  Sum6 : Sum  Orientation=left  Inputs=|+-  SaturateOnIntegerOverflow=on
  Sum7 : Sum  Orientation=left  Inputs=+-|  SaturateOnIntegerOverflow=on
  Sum8 : Sum  Orientation=left  Inputs=++  SaturateOnIntegerOverflow=on
  Sum9 : Sum  Inputs=++|  SaturateOnIntegerOverflow=on
  Switch : Switch  Orientation=left  Threshold=1e-10
  Switch1 : Switch  Orientation=left  Threshold=.5
  Switch2 : Switch  Orientation=left  Threshold=-.5
  Switch3 : Switch  Threshold=Tol
  Terminator1 : Terminator
  Unit Delay : UnitDelay  X0=x0*rand(n*(m+p),1)  SampleTime=T
  vrmult : smxl/Real Matrices/vrmult  dims=[n m m]
  vrmult1 : smxl/Real Matrices/vrmult  dims=[n m m]
  vrmult10 : smxl/Real Matrices/vrmult  Orientation=left  dims=[m m m]
  vrmult2 : smxl/Real Matrices/vrmult  dims=[n m n]
  vrmult3 : smxl/Real Matrices/vrmult  dims=[n m n]
  vrmult4 : smxl/Real Matrices/vrmult  dims=[n n 1]
  vrmult5 : smxl/Real Matrices/vrmult  dims=[n n 1]
  vrmult6 : smxl/Real Matrices/vrmult  Orientation=left  dims=[m m m]
  vrmult7 : smxl/Real Matrices/vrmult  Orientation=left  dims=[n-1 n n]
  vrmult8 : smxl/Real Matrices/vrmult  Orientation=left  dims=[n-1 n n]
  vrmult9 : smxl/Real Matrices/vrmult  Orientation=left  dims=[n-1 n m+p]
  vrsvd : smxl/Real Matrices/vrsvd  dims=[n m]
  vrtrsp4 : smxl/Real Matrices/vrtrsp  dims=[n m]
  vrtrsp5 : smxl/Real Matrices/vrtrsp  dims=[n m]
  vrtrsp6 : smxl/Real Matrices/vrtrsp  Orientation=left  dims=[m m]
  vrvcomp : smxl/Real Matrices/vrvcomp  dims=[n-1 1 m+p]
  out : Outport  Orientation=left  Port=1
  Xinv : Outport  Orientation=left  Port=2
  wires:
  vrmult10/1 -> Xinv/1
  vrtrsp6/1 -> vrmult10/2
  vrmult6/1 -> vrmult10/1
  Math Function/1 -> vrmult6/2
  vrsvd/3 -> vrtrsp6/1, vrmult6/1, vrmult/2
  Sum8/1 -> vrmult9/1
  in/1 -> vrvcomp/2
  vrmult9/1 -> vrvcomp/1
  vrvcomp/1 -> Unit Delay/1
  Unit Delay/1 -> out/1, vrmult9/2
  vrmult7/1 -> Sum8/2
  vrmult8/1 -> Sum8/1
  vrsvd/2 -> Sum9/2
  WX/1 -> vrmult/1, vrsvd/1
  vrsvd/1 -> Terminator1/1
  Constant15/1 -> Sum9/1
  Product4/1 -> Math Function/1, vrmult1/2
  Diag1/1(Out1) -> vrmult7/2
  Diag/1(Out1) -> vrmult8/2
  Switch2/1 -> Diag1/1(In1)
  Switch1/1 -> Diag/1(In1)
  Constant8/1 -> Switch1/1
  Constant10/1 -> vrmult8/1
  Constant9/1 -> vrmult7/1
  Constant14/1 -> Switch2/1
  Constant11/1 -> Switch1/3
  Constant13/1 -> Switch2/3
  Constant12/1 -> Sum7/1
  MinMax1/1 -> Sum7/2
  Sum7/1 -> Switch2/2, Switch1/2
  Abs/1 -> Switch/2
  Constant5/1 -> Switch/1
  Product3/1 -> MinMax1/1
  Constant7/1 -> Product3/2
  Constant6/1 -> Switch/3
  Sum6/1 -> Abs/1
  MinMax/1 -> Sum6/1
  Product2/1 -> Sum6/2, MinMax/1
  Sum5/1 -> Product2/2
  Constant4/1 -> Sum5/2
  vrmult5/1 -> Sum5/1
  vrmult4/1 -> Product2/1
  Constant3/1 -> vrmult4/2, vrmult5/2
  Product/1 -> vrmult5/1
  Product1/1 -> vrmult4/1
  Constant2/1 -> Product1/2, Product/2
  vrmult2/1 -> Product1/1
  vrmult3/1 -> Product/1
  vrtrsp5/1 -> vrmult3/2
  vrmult/1 -> vrtrsp5/1, vrmult1/1  "B"
  vrmult1/1 -> vrmult3/1, vrtrsp4/1, vrmult2/1
  vrtrsp4/1 -> vrmult2/2
  Sum9/1 -> Math Function1/1, Switch3/2
  Constant16/1 -> Switch3/1
  Constant17/1 -> Switch3/3
  Switch3/1 -> Product4/1
  Math Function1/1 -> Product4/2
  Switch/1 -> Product3/1

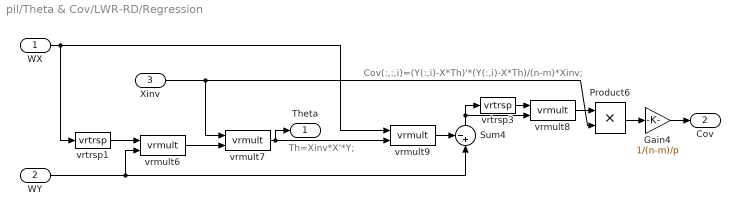
== system pil/Theta & Cov/LWR-RD/Regression ==
  note: Cov(:,:,i)=(Y(:,i)-X*Th)'*(Y(:,i)-X*Th)/(n-m)*Xinv;
  note: Th=Xinv*X'*Y;
  WX : Inport  Port=1  PortWidth=-1  SampleTime=-1  DataType=auto
      settings: SignalType=auto
  WY : Inport  Port=2  PortWidth=-1  SampleTime=-1  DataType=auto
      settings: SignalType=auto
  Xinv : Inport  Port=3  PortWidth=-1  SampleTime=-1  DataType=auto
      settings: SignalType=auto
  Gain4 : Gain  Gain=1/(n-m)/p  SaturateOnIntegerOverflow=on
  Product6 : Product  Inputs=2  SaturateOnIntegerOverflow=on
  Sum4 : Sum  Orientation=up  Inputs=-+|  SaturateOnIntegerOverflow=on
  vrmult6 : smxl/Real Matrices/vrmult  dims=[m n p]
  vrmult7 : smxl/Real Matrices/vrmult  dims=[m m p]
  vrmult8 : smxl/Real Matrices/vrmult  dims=[1 n*p 1]
  vrmult9 : smxl/Real Matrices/vrmult  dims=[n m p]
  vrtrsp1 : smxl/Real Matrices/vrtrsp  dims=[n m]
  vrtrsp3 : smxl/Real Matrices/vrtrsp  dims=[n*p 1]
  Theta : Outport  Port=1
  Cov : Outport  Port=2
  wires:
  vrtrsp1/1 -> vrmult6/1
  WX/1 -> vrtrsp1/1, vrmult9/1
  WY/1 -> vrmult6/2, Sum4/2
  vrtrsp3/1 -> vrmult8/1
  Xinv/1 -> Product6/2, vrmult7/1
  Gain4/1 -> Cov/1
  Product6/1 -> Gain4/1
  vrmult8/1 -> Product6/1
  Sum4/1 -> vrtrsp3/1, vrmult8/2
  vrmult7/1 -> vrmult9/2, Theta/1
  vrmult9/1 -> Sum4/1
  vrmult6/1 -> vrmult7/2

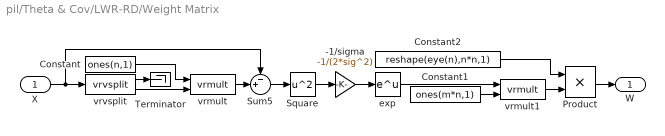
== system pil/Theta & Cov/LWR-RD/Weight Matrix ==
  X : Inport  Port=1  PortWidth=-1  SampleTime=-1  DataType=auto
      settings: SignalType=auto
  -1/sigma : Gain  Gain=-1/(2*sig^2)  SaturateOnIntegerOverflow=on
  Constant : Constant  Value=ones(n,1)
  Constant1 : Constant  Value=ones(m*n,1)
  Constant2 : Constant  Value=reshape(eye(n),n*n,1)
  Product : Product  Inputs=2  SaturateOnIntegerOverflow=on
  Square : Math  Operator=square  OutputSignalType=auto
  Sum5 : Sum  Inputs=-+|  SaturateOnIntegerOverflow=on
  Terminator : Terminator
  exp : Math  Operator=exp  OutputSignalType=auto
  vrmult : smxl/Real Matrices/vrmult  dims=[n 1 m]
  vrmult1 : smxl/Real Matrices/vrmult  dims=[n m n]
  vrvsplit : smxl/Real Matrices/vrvsplit  dims=[n-1 1 m]
  W : Outport  Port=1
  wires:
  X/1 -> vrvsplit/1, Sum5/1
  vrvsplit/1 -> Terminator/1
  vrvsplit/2 -> vrmult/2
  Sum5/1 -> Square/1
  Constant/1 -> vrmult/1
  vrmult/1 -> Sum5/2
  Square/1 -> -1/sigma/1
  -1/sigma/1 -> exp/1
  Product/1 -> W/1
  Constant2/1 -> Product/1
  vrmult1/1 -> Product/2
  Constant1/1 -> vrmult1/2
  exp/1 -> vrmult1/1

== system pil/Theta & Cov/LWR-RD/RD/Diag ==
  In1 : Inport  Orientation=left  Port=1  PortWidth=-1  SampleTime=-1  DataType=auto
      settings: SignalType=auto
  Constant1 : Constant  Orientation=left  Value=ones(n,1)
  Constant8 : Constant  Orientation=left  Value=reshape(eye(n),n*n,1)
  Product4 : Product  Orientation=left  Inputs=2  SaturateOnIntegerOverflow=on
  vrmult6 : smxl/Real Matrices/vrmult  Orientation=left  dims=[n 1 n]
  Out1 : Outport  Orientation=left  Port=1
  wires:
  Product4/1 -> Out1/1
  In1/1 -> vrmult6/2
  Constant8/1 -> Product4/2
  vrmult6/1 -> Product4/1
  Constant1/1 -> vrmult6/1

== system pil/Theta & Cov/LWR-RD/RD/Diag1 ==
  In1 : Inport  Orientation=left  Port=1  PortWidth=-1  SampleTime=-1  DataType=auto
      settings: SignalType=auto
  Constant1 : Constant  Orientation=left  Value=ones(n,1)
  Constant8 : Constant  Orientation=left  Value=reshape(eye(n),n*n,1)
  Product4 : Product  Orientation=left  Inputs=2  SaturateOnIntegerOverflow=on
  vrmult6 : smxl/Real Matrices/vrmult  Orientation=left  dims=[n 1 n]
  Out1 : Outport  Orientation=left  Port=1
  wires:
  Constant1/1 -> vrmult6/1
  vrmult6/1 -> Product4/1
  Constant8/1 -> Product4/2
  In1/1 -> vrmult6/2
  Product4/1 -> Out1/1
